simulink model "ACC_demo"  (R2016a)
settings: Solver=VariableStepAuto  StartTime=0  StopTime=30  MaxStep=0.3  RelTol=1e-5
values from neighbouring files (symbols this model uses):
  gearRatio = 15.0    [ACC_dict.sldd]
  initialVelocity = 0.0    [ACC_dict.sldd]
  rollingRadius = 0.3    [ACC_dict.sldd]
libraries: fl_lib x37, nesl_utility x28, sdl_lib x20, sh_lib x7, simulink x1
settings Model: DataDictionary=ACC_dict.sldd  FPTRunName=FPA_Reference  PauseTimes=3  Creator=oskar  LastModifiedBy=Oskar
settings SolverCC: AlgebraicLoopSolver=LineSearch  SolverResetMethod=Robust
settings DataIOCC: SaveFormat=StructureWithTime  ReturnWorkspaceOutputs=on  ReturnWorkspaceOutputsName=spidata
settings HardwareCC: ProdBitPerLong=64  ProdLargestAtomicInteger=Long  ProdLargestAtomicFloat=Double  ProdLongLongMode=on  ProdHWDeviceType=Intel->x86-64  TargetBitPerLong=64  TargetBitPerPointer=64  TargetLongLongMode=on  TargetIntDivRoundTo=Zero  TargetEndianess=LittleEndian  TargetWordSize=64  TargetHWDeviceType=MATLAB Host  ProdEqTarget=off
settings SFSimCC: SimUserSources=protocol.c
settings RTWCC: SystemTargetFile=rsim.tlc  TemplateMakefile=rsim_default_tmf  Description=Rapid Simulation Target  RTWUseSimCustomCode=on  CustomSource=protocol.c  RTWCompilerOptimization=on
settings CodeAppCC: MaxIdLength=95
settings RSimTargetCC: ERTMultiwordTypeDef=System defined  ERTMultiwordLength=256  GeneratePreprocessorConditionals=Use local settings
settings SimscapeCC: SimscapeLogSimulationStatistics=on  SimscapeLogLimitData=off

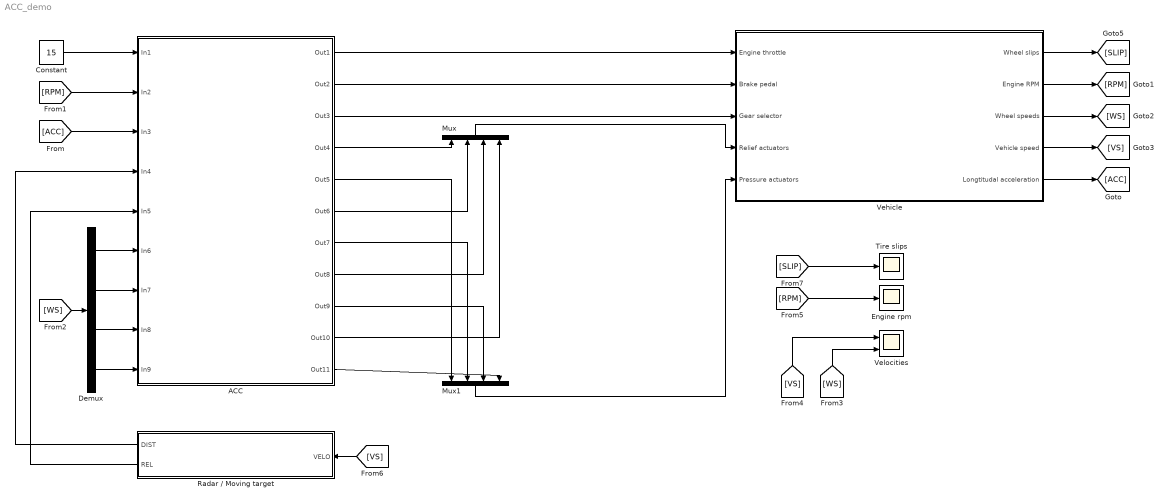
== system ACC_demo ==
  ACC : Subsystem  mask(ARSim){simPath='/Users/Oskar/dev/autosar/arsim-examples/dist/build/acc/acc', numInput=9, numOutput=11}
      mask prompts: simPath "Simulator path"; numInput "# input ports"; numOutput "# output ports"
      mask help:
      | This component acts as an S-function wrapper for the ARSim component. The simulator path parameter needs to be configured as a string pointing to the location of the compiled AUTOSAR component (i.e. with simulateUsingExternal).
      |
      | When the model is initialized, the AUTOSAR simulator will ask for specific port widths. This cannot be adjusted automatically by the Simulink component (yet), so manual intervention is needed, hence the # input/output ports dialogs.
      mask Display: ;port_label('input', 1, 'CRUISE');port_label('input', 2, 'RPM');port_label('input', 3, 'ACCEL');port_label('input', 4, 'DIST');port_label('input', 5, 'REL');port_label('input', 6, 'WHEEL1');port_label('input', 7, 'WHEEL2');port_label('input', 8, 'WHEEL3');port_label('input', 9, 'WHEEL4');port_label('output', 1, 'THR_OUT');port_label('output', 2, 'BRK_OUT');port_label('output', 3, 'GEAR');port_label('output', 4, 'RE');port_label('output', 5, 'PR');port_label('output', 6, 'RE');port_label('output', 7, 'PR');port_label('output', 8, 'RE');port_label('output', 9, 'PR');port_label('output', 10, 'RE');port_label('output', 11, 'PR')
  Constant : Constant  Value=15
  Demux : Demux
  Engine rpm : Scope
  Mux : Mux
  Mux1 : Mux
  Radar / Moving target : Subsystem  mask{dist0=50, velo0=10}
      mask prompts: dist0 "Initial distance"; velo0 "Initial velocity"
  Tire slips : Scope
  Vehicle : Subsystem
  Velocities : Scope  NumInputPorts=2
  wires:
  ACC/4(Out4) -> Mux/1
  ACC/6(Out6) -> Mux/2
  ACC/8(Out8) -> Mux/3
  ACC/10(Out10) -> Mux/4
  ACC/5(Out5) -> Mux1/1
  ACC/7(Out7) -> Mux1/2
  ACC/9(Out9) -> Mux1/3
  ACC/11(Out11) -> Mux1/4
  ACC/1(Out1) -> Vehicle/1(Engine throttle)
  ACC/2(Out2) -> Vehicle/2(Brake pedal)
  ACC/3(Out3) -> Vehicle/3(Gear selector)
  Mux/1 -> Vehicle/4(Relief actuators)
  Mux1/1 -> Vehicle/5(Pressure actuators)
  [ACC] -> ACC/3(In3)
  Vehicle/5(Longtitudal acceleration) -> [ACC]
  Vehicle/2(Engine RPM) -> [RPM]
  [RPM] -> ACC/2(In2)
  Constant/1 -> ACC/1(In1)
  [WS] -> Demux/1
  [WS] -> Velocities/2
  Vehicle/4(Vehicle speed) -> [VS]
  [VS] -> Velocities/1
  [RPM] -> Engine rpm/1
  [SLIP] -> Tire slips/1
  Vehicle/1(Wheel slips) -> [SLIP]
  Vehicle/3(Wheel speeds) -> [WS]
  Radar / Moving target/1(DIST) -> ACC/4(In4)
  Demux/1 -> ACC/6(In6)
  Demux/2 -> ACC/7(In7)
  Demux/3 -> ACC/8(In8)
  Demux/4 -> ACC/9(In9)
  Radar / Moving target/2(REL) -> ACC/5(In5)
  [VS] -> Radar / Moving target/1(VELO)

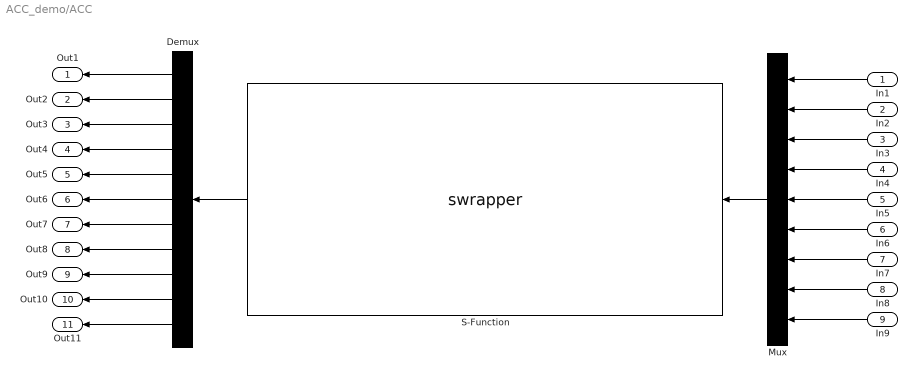
== system ACC_demo/ACC ==
  In1 : Inport  PortDimensions=1
  In2 : Inport  Port=2  PortDimensions=1
  In3 : Inport  Port=3  PortDimensions=1
  In4 : Inport  Port=4  PortDimensions=1
  In5 : Inport  Port=5  PortDimensions=1
  In6 : Inport  Port=6  PortDimensions=1
  In7 : Inport  Port=7  PortDimensions=1
  In8 : Inport  Port=8  PortDimensions=1
  In9 : Inport  Port=9  PortDimensions=1
  Demux : Demux  Outputs=numOutput
  Mux : Mux  Inputs=numInput
  S-Function : S-Function  FunctionName=swrapper  Parameters=simPath  SFunctionDeploymentMode=off  EnableBusSupport=off
  Out1 : Outport  PortDimensions=1
  Out2 : Outport  Port=2  PortDimensions=1
  Out3 : Outport  Port=3  PortDimensions=1
  Out4 : Outport  Port=4  PortDimensions=1
  Out5 : Outport  Port=5  PortDimensions=1
  Out6 : Outport  Port=6  PortDimensions=1
  Out7 : Outport  Port=7  PortDimensions=1
  Out8 : Outport  Port=8  PortDimensions=1
  Out9 : Outport  Port=9  PortDimensions=1
  Out10 : Outport  Port=10  PortDimensions=1
  Out11 : Outport  Port=11  PortDimensions=1
  wires:
  In1/1 -> Mux/1
  Mux/1 -> S-Function/1
  In2/1 -> Mux/2
  S-Function/1 -> Demux/1
  Demux/1 -> Out1/1
  Demux/2 -> Out2/1
  In3/1 -> Mux/3
  In4/1 -> Mux/4
  In5/1 -> Mux/5
  In6/1 -> Mux/6
  Demux/3 -> Out3/1
  In7/1 -> Mux/7
  Demux/11 -> Out11/1
  Demux/10 -> Out10/1
  Demux/9 -> Out9/1
  Demux/8 -> Out8/1
  Demux/7 -> Out7/1
  Demux/6 -> Out6/1
  Demux/5 -> Out5/1
  Demux/4 -> Out4/1
  In8/1 -> Mux/8
  In9/1 -> Mux/9

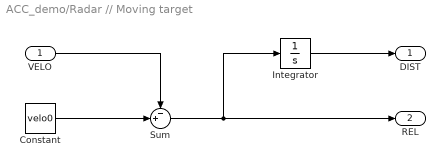
== system ACC_demo/Radar // Moving target ==
  VELO : Inport
  Constant : Constant  Value=velo0
  Integrator : Integrator  InitialCondition=dist0
  Sum : Sum  Inputs=-+|
  DIST : Outport
  REL : Outport  Port=2
  wires:
  Integrator/1 -> DIST/1
  VELO/1 -> Sum/1
  Constant/1 -> Sum/2
  Sum/1 -> Integrator/1, REL/1

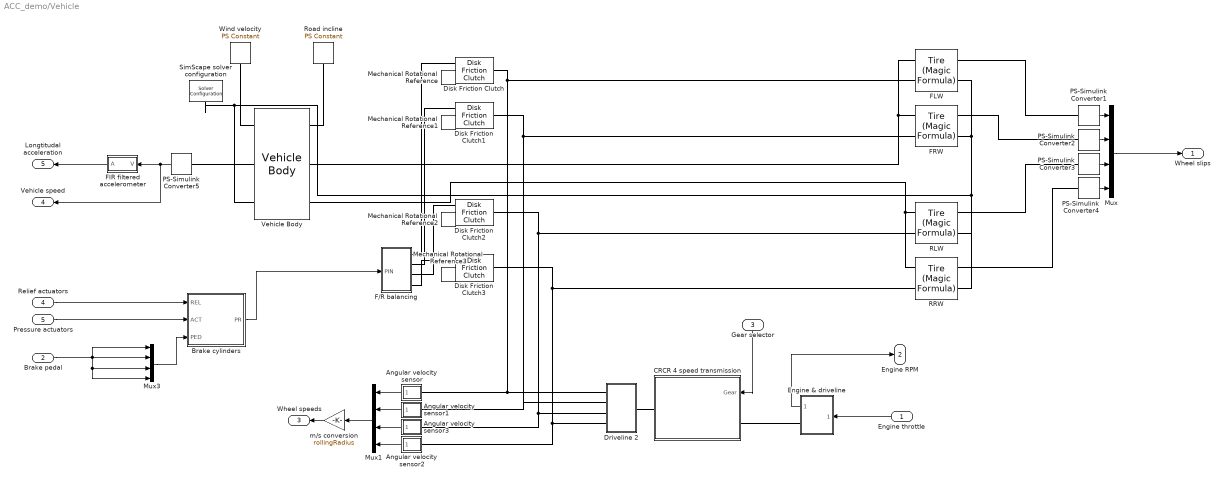
== system ACC_demo/Vehicle ==
  Engine throttle : Inport
  Brake pedal : Inport  Port=2
  Gear selector : Inport  Port=3
  Relief actuators : Inport  Port=4
  Pressure actuators : Inport  Port=5
  Angular velocity sensor : Subsystem
  Angular velocity sensor1 : Subsystem
  Angular velocity sensor2 : Subsystem
  Angular velocity sensor3 : Subsystem
  Brake cylinders : Subsystem  TreatAsAtomicUnit=on
  CRCR 4 speed transmission : Subsystem  mask{ShowInLibBrowser=0}
      settings: OpenFcn=open_system(gcb,'force');
  Disk Friction Clutch{,1..3} (4 alike) : sdl_lib/Clutches/Disk Friction Clutch  geometry_model=1  r_eff=torqueRadius mm  d_o=150 mm  d_i=100 mm  nS=numSurf  piston_area=pistonArea m^2  unidirectional=0  friction_model=1  mu_coulomb=clutchKineticF  mu_w_vector=[ 0 0.1 0.2 0.3 0.4 0.5 1 2 5 10 100 1000 ] rad/s  mu_coulomb_vector=[ 0.29 0.28 0.26 0.22 0.21 0.2 0.2 0.19 0.19 0.19 0.19 0.19 ]  mu_interp_method=1  mu_extrap_method=1  mu_static=clutchStaticF  d_f=1  w_tol=clutchVeloTolRads rad/s  pressure_min=clutchPressureTresh Pa  mu_visc=0 N*m/(rad/s)  initial_state_locked=0
  Driveline 2 : Subsystem
  Engine & driveline : Subsystem
  F/R balancing : Subsystem  mask(F/R Balance){RGain=0.7}
      mask prompts: RGain "Rear pressure gain"
      mask help: Scale the amount of pressure directed to the rear wheels by a constant factor (default 0.7).
  FIR filtered accelerometer : Subsystem
  FLW : sdl_lib/Tires & Vehicles/Tire (Magic Formula)  parameterization=1  F_z1=3e+3 N  F_x1=3.5e+3 N  kappa1=10  B_m=10  C_m=1.9  D_m=1  E_m=0.97  fz0=4e+3 N  p_Cx=1.685  p_Dx=[ 1.21 -0.037 ]  p_Ex=[ 0.344 0.095 -0.02 0 ]  p_Kx=[ 21.51 -0.163 0.245 ]  p_Hx=[ -0.002 0.002 ]  p_Vx=[ 0 0 ]  v_tr_thr=0.1 m/s  r_e=rollingRadius m  model_compliance=0  stiffness=1e+6 N/m  damping=1000 N/(m/s)  model_inertia=0  inertia=1 kg*m^2  initial_velocity=0 rad/s  model_resistance=0  resistance_model=1  coeff=0.015  p_tire=250e3 Pa  alpha=-0.003  beta=0.97  coeff_a=84e-4  coeff_b=6.2e-4 s/m  coeff_c=1.6e-4 s^2/m^2  v_thr=1e-3 m/s
  FRW : sdl_lib/Tires & Vehicles/Tire (Magic Formula)  parameterization=1  F_z1=3e+3 N  F_x1=3.5e+3 N  kappa1=10  B_m=10  C_m=1.9  D_m=1  E_m=0.97  fz0=4e+3 N  p_Cx=1.685  p_Dx=[ 1.21 -0.037 ]  p_Ex=[ 0.344 0.095 -0.02 0 ]  p_Kx=[ 21.51 -0.163 0.245 ]  p_Hx=[ -0.002 0.002 ]  p_Vx=[ 0 0 ]  v_tr_thr=0.1 m/s  r_e=rollingRadius m  model_compliance=0  stiffness=1e+6 N/m  damping=1000 N/(m/s)  model_inertia=0  inertia=1 kg*m^2  initial_velocity=0 rad/s  model_resistance=0  resistance_model=1  coeff=0.015  p_tire=250e3 Pa  alpha=-0.003  beta=0.97  coeff_a=84e-4  coeff_b=6.2e-4 s/m  coeff_c=1.6e-4 s^2/m^2  v_thr=1e-3 m/s
  Mechanical Rotational Reference{,1..3} (4 alike) : fl_lib/Mechanical/Rotational Elements/Mechanical Rotational Reference
  Mux : Mux
  Mux1 : Mux
  Mux3 : Mux
  PS-Simulink Converter{1..5} (5 alike) : nesl_utility/PS-Simulink Converter  PhysicalDomain=network_engine_domain  SubClassName=ps_output  LeftPortType=input  RightPortType=output  PseudoPeriodic=off  Frequencies=[]  Unit=1  AffineConversion=off
  RLW : sdl_lib/Tires & Vehicles/Tire (Magic Formula)  parameterization=1  F_z1=3e+3 N  F_x1=3.5e+3 N  kappa1=10  B_m=10  C_m=1.9  D_m=1  E_m=0.97  fz0=4e+3 N  p_Cx=1.685  p_Dx=[ 1.21 -0.037 ]  p_Ex=[ 0.344 0.095 -0.02 0 ]  p_Kx=[ 21.51 -0.163 0.245 ]  p_Hx=[ -0.002 0.002 ]  p_Vx=[ 0 0 ]  v_tr_thr=0.1 m/s  r_e=rollingRadius m  model_compliance=0  stiffness=1e+6 N/m  damping=1000 N/(m/s)  model_inertia=0  inertia=1 kg*m^2  initial_velocity=0 rad/s  model_resistance=0  resistance_model=1  coeff=0.015  p_tire=250e3 Pa  alpha=-0.003  beta=0.97  coeff_a=84e-4  coeff_b=6.2e-4 s/m  coeff_c=1.6e-4 s^2/m^2  v_thr=1e-3 m/s
  RRW : sdl_lib/Tires & Vehicles/Tire (Magic Formula)  parameterization=1  F_z1=3e+3 N  F_x1=3.5e+3 N  kappa1=10  B_m=10  C_m=1.9  D_m=1  E_m=0.97  fz0=4e+3 N  p_Cx=1.685  p_Dx=[ 1.21 -0.037 ]  p_Ex=[ 0.344 0.095 -0.02 0 ]  p_Kx=[ 21.51 -0.163 0.245 ]  p_Hx=[ -0.002 0.002 ]  p_Vx=[ 0 0 ]  v_tr_thr=0.1 m/s  r_e=rollingRadius m  model_compliance=0  stiffness=1e+6 N/m  damping=1000 N/(m/s)  model_inertia=0  inertia=1 kg*m^2  initial_velocity=0 rad/s  model_resistance=0  resistance_model=1  coeff=0.015  p_tire=250e3 Pa  alpha=-0.003  beta=0.97  coeff_a=84e-4  coeff_b=6.2e-4 s/m  coeff_c=1.6e-4 s^2/m^2  v_thr=1e-3 m/s
  Road incline : fl_lib/Physical Signals/Sources/PS Constant  constant=0
  SimScape solver configuration : nesl_utility/Solver Configuration  PhysicalDomain=network_engine_domain  SubClassName=solver  LeftPortType=input  RightPortType=generic  Accelerate=off  Tones=[]  Harmonics=[]  SimulateNoise=off  Profile=off  UseLocalSampling=off  EnableSwitchedLinearOptims=on  FrequencyDomain=off  UseCCode=off  RelTol=0.001  AbsTol=1e-06  MinStep=1e-09  ToWorkspace=off  RevertToSquareIcSolve=off  NumHomotopyIterations=100  PhasorMode=off  PhasorModeNumHarmonics=1  OverrideAbsTol=off  DoDC=off  ResidualTolerance=1e-09  UseLocalSolver=off  LocalSolverChoice=NE_TRAPEZOIDAL_ADVANCER  LocalSolverSampleTime=0.001  DoFixedCost=off  MaxNonlinIter=3  MaxModeIter=2  LinearAlgebra=Sparse  DelaysMemoryBudget=1024  AutomaticFiltering=on  FilteringTimeConstant=0.001
  Vehicle Body : sdl_lib/Tires & Vehicles/Vehicle Body  mass=1500 kg  n_w=2  x_f=1.4 m  x_r=1.6 m  y_c=0.5 m  area=4 m^2  Cd=0.4  v0=initialVelocity m/s
  Wind velocity : fl_lib/Physical Signals/Sources/PS Constant  constant=10
  m/s conversion : Gain  Gain=rollingRadius
  Wheel slips : Outport
  Engine RPM : Outport  Port=2
  Wheel speeds : Outport  Port=3
  Vehicle speed : Outport  Port=4
  Longtitudal acceleration : Outport  Port=5
  wires:
  m/s conversion/1 -> Wheel speeds/1
  PS-Simulink Converter4/1 -> Mux/4
  PS-Simulink Converter1/1 -> Mux/1
  Mux/1 -> Wheel slips/1
  PS-Simulink Converter2/1 -> Mux/2
  PS-Simulink Converter3/1 -> Mux/3
  Pressure actuators/1 -> Brake cylinders/2(ACT)
  Mux1/1 -> m/s conversion/1
  Engine throttle/1 -> Engine & driveline/1(Throttle)
  Relief actuators/1 -> Brake cylinders/1(REL)
  Angular velocity sensor/1(Out1) -> Mux1/1
  Angular velocity sensor3/1(Out1) -> Mux1/3
  Angular velocity sensor1/1(Out1) -> Mux1/2
  Angular velocity sensor2/1(Out1) -> Mux1/4
  Mux3/1 -> Brake cylinders/3(PED)
  Brake pedal/1 -> Mux3/4, Mux3/3, Mux3/2, Mux3/1
  Brake cylinders/1(PR) -> F/R balancing/1(PIN)
  Engine & driveline/1(rpm) -> Engine RPM/1
  Gear selector/1 -> CRCR 4 speed transmission/1(Gear)
  FIR filtered accelerometer/1(A) -> Longtitudal acceleration/1
  PS-Simulink Converter5/1 -> Vehicle speed/1, FIR filtered accelerometer/1(V)
  connections:
  PS-Simulink Converter4/LConn1 -- RRW/RConn1
  CRCR 4 speed transmission/RConn1 -- Driveline 2/RConn1
  PS-Simulink Converter3/LConn1 -- RLW/RConn1
  PS-Simulink Converter2/LConn1 -- FRW/RConn1
  PS-Simulink Converter1/LConn1 -- FLW/RConn1
  Vehicle Body/RConn1 -- RRW/LConn1 -- RLW/LConn1
  Vehicle Body/RConn2 -- FLW/LConn1 -- FRW/LConn1
  Wind velocity/RConn1 -- Vehicle Body/LConn3
  Vehicle Body/LConn1 -- FLW/RConn2 -- FRW/RConn2 -- RLW/RConn2 -- RRW/RConn2 -- SimScape solver configuration/RConn1
  Road incline/RConn1 -- Vehicle Body/RConn3
  Angular velocity sensor3/LConn1 -- Driveline 2/LConn3 -- Disk Friction Clutch2/RConn1 -- RLW/LConn2
  Disk Friction Clutch1/RConn1 -- Angular velocity sensor1/LConn1 -- Driveline 2/LConn2 -- FRW/LConn2
  Angular velocity sensor/LConn1 -- Disk Friction Clutch/RConn1 -- FLW/LConn2 -- Driveline 2/LConn1
  Angular velocity sensor2/LConn1 -- Driveline 2/LConn4 -- Disk Friction Clutch3/RConn1 -- RRW/LConn2
  Mechanical Rotational Reference/LConn1 -- Disk Friction Clutch/LConn2
  Mechanical Rotational Reference2/LConn1 -- Disk Friction Clutch2/LConn2
  Mechanical Rotational Reference1/LConn1 -- Disk Friction Clutch1/LConn2
  Mechanical Rotational Reference3/LConn1 -- Disk Friction Clutch3/LConn2
  Disk Friction Clutch/LConn1 -- F/R balancing/RConn1
  Disk Friction Clutch1/LConn1 -- F/R balancing/RConn2
  Disk Friction Clutch2/LConn1 -- F/R balancing/RConn3
  Disk Friction Clutch3/LConn1 -- F/R balancing/RConn4
  Engine & driveline/RConn1 -- CRCR 4 speed transmission/LConn1
  PS-Simulink Converter5/LConn1 -- Vehicle Body/LConn2

== system ACC_demo/Vehicle/Angular velocity sensor ==
  PS-Simulink Converter3 : nesl_utility/PS-Simulink Converter  PhysicalDomain=network_engine_domain  SubClassName=ps_output  LeftPortType=input  RightPortType=output  PseudoPeriodic=off  Frequencies=[]  Unit=1  AffineConversion=off
  Reference : fl_lib/Mechanical/Rotational Elements/Mechanical Rotational Reference
  Rotational Motion Sensor : fl_lib/Mechanical/Mechanical Sensors/Ideal Rotational Motion Sensor  offset=0 rad
  Axle : PMIOPort  Port=1  Side=Left
  Out1 : Outport
  wires:
  PS-Simulink Converter3/1 -> Out1/1
  connections:
  Axle/RConn1 -- Rotational Motion Sensor/LConn1
  Reference/LConn1 -- Rotational Motion Sensor/RConn1
  Rotational Motion Sensor/RConn2 -- PS-Simulink Converter3/LConn1

== system ACC_demo/Vehicle/Angular velocity sensor1 ==
  PS-Simulink Converter3 : nesl_utility/PS-Simulink Converter  PhysicalDomain=network_engine_domain  SubClassName=ps_output  LeftPortType=input  RightPortType=output  PseudoPeriodic=off  Frequencies=[]  Unit=1  AffineConversion=off
  Reference : fl_lib/Mechanical/Rotational Elements/Mechanical Rotational Reference
  Rotational Motion Sensor : fl_lib/Mechanical/Mechanical Sensors/Ideal Rotational Motion Sensor  offset=0 rad
  Axle : PMIOPort  Port=1  Side=Left
  Out1 : Outport
  wires:
  PS-Simulink Converter3/1 -> Out1/1
  connections:
  Axle/RConn1 -- Rotational Motion Sensor/LConn1
  Reference/LConn1 -- Rotational Motion Sensor/RConn1
  Rotational Motion Sensor/RConn2 -- PS-Simulink Converter3/LConn1

== system ACC_demo/Vehicle/Angular velocity sensor2 ==
  PS-Simulink Converter3 : nesl_utility/PS-Simulink Converter  PhysicalDomain=network_engine_domain  SubClassName=ps_output  LeftPortType=input  RightPortType=output  PseudoPeriodic=off  Frequencies=[]  Unit=1  AffineConversion=off
  Reference : fl_lib/Mechanical/Rotational Elements/Mechanical Rotational Reference
  Rotational Motion Sensor : fl_lib/Mechanical/Mechanical Sensors/Ideal Rotational Motion Sensor  offset=0 rad
  Axle : PMIOPort  Port=1  Side=Left
  Out1 : Outport
  wires:
  PS-Simulink Converter3/1 -> Out1/1
  connections:
  Axle/RConn1 -- Rotational Motion Sensor/LConn1
  Reference/LConn1 -- Rotational Motion Sensor/RConn1
  Rotational Motion Sensor/RConn2 -- PS-Simulink Converter3/LConn1

== system ACC_demo/Vehicle/Angular velocity sensor3 ==
  PS-Simulink Converter3 : nesl_utility/PS-Simulink Converter  PhysicalDomain=network_engine_domain  SubClassName=ps_output  LeftPortType=input  RightPortType=output  PseudoPeriodic=off  Frequencies=[]  Unit=1  AffineConversion=off
  Reference : fl_lib/Mechanical/Rotational Elements/Mechanical Rotational Reference
  Rotational Motion Sensor : fl_lib/Mechanical/Mechanical Sensors/Ideal Rotational Motion Sensor  offset=0 rad
  Axle : PMIOPort  Port=1  Side=Left
  Out1 : Outport
  wires:
  PS-Simulink Converter3/1 -> Out1/1
  connections:
  Axle/RConn1 -- Rotational Motion Sensor/LConn1
  Reference/LConn1 -- Rotational Motion Sensor/RConn1
  Rotational Motion Sensor/RConn2 -- PS-Simulink Converter3/LConn1

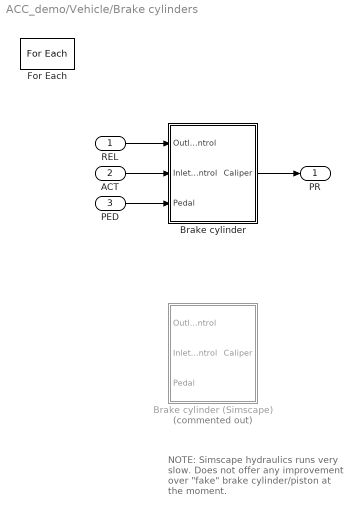
== system ACC_demo/Vehicle/Brake cylinders ==
  note: NOTE: Simscape hydraulics
      | runs very slow. Does not offer
      | any improvement over "fake"
      | brake cylinder/piston at the
      | moment.
  REL : Inport  Partition=on  PartitionDimension=1  PartitionWidth=1
  ACT : Inport  Port=2  Partition=on  PartitionDimension=1  PartitionWidth=1
  PED : Inport  Port=3  Partition=on  PartitionDimension=1  PartitionWidth=1
  Brake cylinder : Subsystem
  Brake cylinder (Simscape) : Subsystem  Commented=on
  For Each : ForEach  DisableCoverage=on  IndexMode=One-based
  PR : Outport  Unit=Pa  ConcatenationDimension=1
  wires:
  Brake cylinder/1(Caliper) -> PR/1
  REL/1 -> Brake cylinder/1(Outlet control)
  ACT/1 -> Brake cylinder/2(Inlet control)
  PED/1 -> Brake cylinder/3(Pedal)

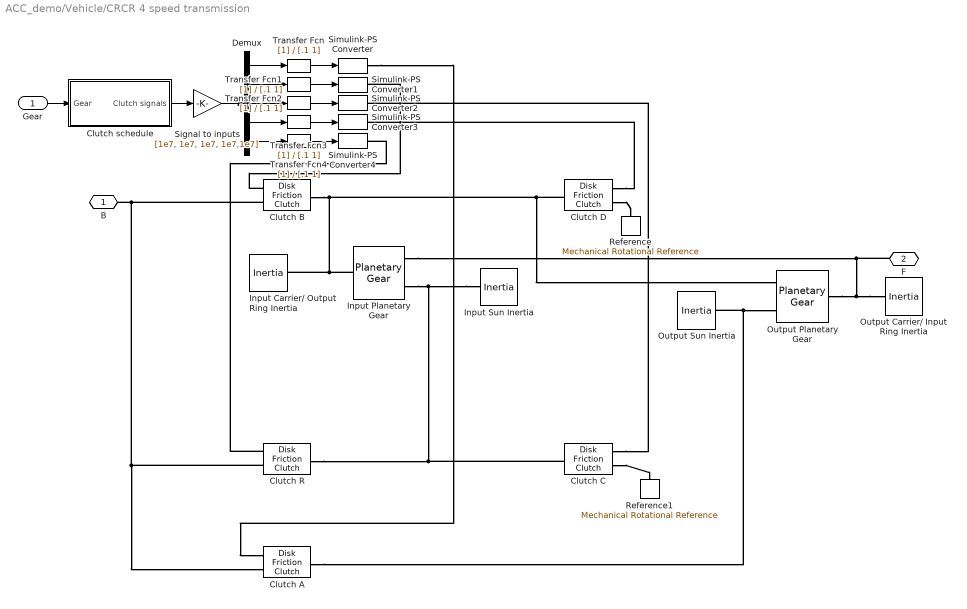
== system ACC_demo/Vehicle/CRCR 4 speed transmission ==
  Gear : Inport
  Clutch A : sdl_lib/Clutches/Disk Friction Clutch  geometry_model=1  r_eff=.05 m  d_o=0.15 m  d_i=0.1 m  nS=6  piston_area=1e-3 m^2  unidirectional=0  friction_model=1  mu_coulomb=.5  mu_w_vector=[ 0 0.1 0.2 0.3 0.4 0.5 1 2 5 10 100 1000 ] rad/s  mu_coulomb_vector=[ 0.29 0.28 0.26 0.22 0.21 0.2 0.2 0.19 0.19 0.19 0.19 0.19 ]  mu_interp_method=1  mu_extrap_method=1  mu_static=.55  d_f=1  w_tol=1e-3 rad/s  pressure_min=1e4 Pa  mu_visc=0 N*m/(rad/s)  initial_state_locked=1
  Clutch B : sdl_lib/Clutches/Disk Friction Clutch  geometry_model=1  r_eff=.05 m  d_o=0.15 m  d_i=0.1 m  nS=6  piston_area=1e-3 m^2  unidirectional=0  friction_model=1  mu_coulomb=.5  mu_w_vector=[ 0 0.1 0.2 0.3 0.4 0.5 1 2 5 10 100 1000 ] rad/s  mu_coulomb_vector=[ 0.29 0.28 0.26 0.22 0.21 0.2 0.2 0.19 0.19 0.19 0.19 0.19 ]  mu_interp_method=1  mu_extrap_method=1  mu_static=.55  d_f=1  w_tol=1e-3 rad/s  pressure_min=1e4 Pa  mu_visc=0 N*m/(rad/s)  initial_state_locked=0
  Clutch C : sdl_lib/Clutches/Disk Friction Clutch  geometry_model=1  r_eff=.05 m  d_o=0.15 m  d_i=0.1 m  nS=6  piston_area=1e-3 m^2  unidirectional=0  friction_model=1  mu_coulomb=.5  mu_w_vector=[ 0 0.1 0.2 0.3 0.4 0.5 1 2 5 10 100 1000 ] rad/s  mu_coulomb_vector=[ 0.29 0.28 0.26 0.22 0.21 0.2 0.2 0.19 0.19 0.19 0.19 0.19 ]  mu_interp_method=1  mu_extrap_method=1  mu_static=.55  d_f=1  w_tol=1e-3 rad/s  pressure_min=1e4 Pa  mu_visc=0 N*m/(rad/s)  initial_state_locked=0
  Clutch D : sdl_lib/Clutches/Disk Friction Clutch  geometry_model=1  r_eff=.05 m  d_o=0.15 m  d_i=0.1 m  nS=6  piston_area=1e-3 m^2  unidirectional=0  friction_model=1  mu_coulomb=.5  mu_w_vector=[ 0 0.1 0.2 0.3 0.4 0.5 1 2 5 10 100 1000 ] rad/s  mu_coulomb_vector=[ 0.29 0.28 0.26 0.22 0.21 0.2 0.2 0.19 0.19 0.19 0.19 0.19 ]  mu_interp_method=1  mu_extrap_method=1  mu_static=.55  d_f=1  w_tol=1e-3 rad/s  pressure_min=1e4 Pa  mu_visc=0 N*m/(rad/s)  initial_state_locked=1
  Clutch R : sdl_lib/Clutches/Disk Friction Clutch  geometry_model=1  r_eff=.05 m  d_o=0.15 m  d_i=0.1 m  nS=6  piston_area=1e-3 m^2  unidirectional=0  friction_model=1  mu_coulomb=.5  mu_w_vector=[ 0 0.1 0.2 0.3 0.4 0.5 1 2 5 10 100 1000 ] rad/s  mu_coulomb_vector=[ 0.29 0.28 0.26 0.22 0.21 0.2 0.2 0.19 0.19 0.19 0.19 0.19 ]  mu_interp_method=1  mu_extrap_method=1  mu_static=.55  d_f=1  w_tol=1e-3 rad/s  pressure_min=1e4 Pa  mu_visc=0 N*m/(rad/s)  initial_state_locked=0
  Clutch schedule : Subsystem
  Demux : Demux  Outputs=5
  "Input Planetary Gear " : sdl_lib/Gears/Planetary Gear  rs_ratio=2  friction_model=1  efficiency=[ 0.96 0.98 ]  mu_visc=[ 0 0 ] N*m/(rad/s)  pwr_thr=[ 0.001 0.001 ] W  planet_inertia=0 kg*m^2  temperature_TLU=[ 280 300 320 ] K  efficiency_sp_TLU=[ 0.95 0.9 0.85 ]  efficiency_rp_TLU=[ 0.95 0.9 0.85 ]  thermal_mass=50 J/K  T_init=300 K
  Input Sun Inertia : fl_lib/Mechanical/Rotational Elements/Inertia  inertia=1e-4 kg*m^2  w_specify=on  w_priority=High  w=0 rad/s  t_specify=off  t_priority=High  t=0 N*m
  Input Carrier/ Output Ring Inertia : fl_lib/Mechanical/Rotational Elements/Inertia  inertia=1e-4 kg*m^2  w_specify=off  w_priority=High  w=initialVelocity/rollingRadius rad/s  t_specify=off  t_priority=High  t=0 N*m
  Output Planetary Gear : sdl_lib/Gears/Planetary Gear  rs_ratio=2  friction_model=1  efficiency=[ 0.96 0.98 ]  mu_visc=[ 0 0 ] N*m/(rad/s)  pwr_thr=[ 0.001 0.001 ] W  planet_inertia=0 kg*m^2  temperature_TLU=[ 280 300 320 ] K  efficiency_sp_TLU=[ 0.95 0.9 0.85 ]  efficiency_rp_TLU=[ 0.95 0.9 0.85 ]  thermal_mass=50 J/K  T_init=300 K
  Output Sun Inertia : fl_lib/Mechanical/Rotational Elements/Inertia  inertia=1e-4 kg*m^2  w_specify=on  w_priority=High  w=3*gearRatio*initialVelocity/rollingRadius rad/s  t_specify=off  t_priority=High  t=0 N*m
  "Output Carrier/ Input Ring Inertia " : fl_lib/Mechanical/Rotational Elements/Inertia  inertia=1e-4 kg*m^2  w_specify=on  w_priority=Low  w=gearRatio*initialVelocity/rollingRadius rad/s  t_specify=off  t_priority=High  t=0 N*m
  Reference : fl_lib/Mechanical/Rotational Elements/Mechanical Rotational Reference
  Reference1 : fl_lib/Mechanical/Rotational Elements/Mechanical Rotational Reference
  Signal to inputs : Gain  Gain=[1e7, 1e7, 1e7, 1e7,1e7]
  Simulink-PS Converter{,1..4} (5 alike) : nesl_utility/Simulink-PS Converter  PhysicalDomain=network_engine_domain  SubClassName=ps_input  LeftPortType=input  RightPortType=output  PseudoPeriodic=off  Frequencies=[]  NoiseDistribution=none  NoiseParameters=[]  Unit=1  AffineConversion=off  InputFiltering=off  SimscapeFilterOrder=1  InputFilterTimeConstant=0.001  UdotUserProvided=1
  Transfer Fcn{,1..4} (5 alike) : TransferFcn  Denominator=[.1 1]
  B : PMIOPort  Port=1  Side=Left
  F : PMIOPort  Port=2  Side=Right
  wires:
  Transfer Fcn1/1 -> Simulink-PS Converter1/1
  Transfer Fcn2/1 -> Simulink-PS Converter2/1
  Transfer Fcn3/1 -> Simulink-PS Converter3/1
  Transfer Fcn4/1 -> Simulink-PS Converter4/1
  Demux/4 -> Transfer Fcn3/1
  Demux/5 -> Transfer Fcn4/1
  Demux/3 -> Transfer Fcn2/1
  Demux/2 -> Transfer Fcn1/1
  Transfer Fcn/1 -> Simulink-PS Converter/1
  Gear/1 -> Clutch schedule/1(Gear)
  Clutch schedule/1(Clutch signals) -> Signal to inputs/1
  Signal to inputs/1 -> Demux/1
  Demux/1 -> Transfer Fcn/1
  connections:
  "Output Carrier/ Input Ring Inertia "/LConn1 -- "Input Planetary Gear "/RConn1 -- F/RConn1 -- Output Planetary Gear/LConn1
  Output Sun Inertia/LConn1 -- Clutch A/RConn1 -- Output Planetary Gear/RConn2
  Input Sun Inertia/LConn1 -- "Input Planetary Gear "/RConn2 -- Clutch C/RConn1 -- Clutch R/RConn1
  Input Carrier/ Output Ring Inertia/LConn1 -- "Input Planetary Gear "/LConn1 -- Clutch B/RConn1 -- Clutch D/RConn1 -- Output Planetary Gear/RConn1
  Clutch R/LConn2 -- Clutch A/LConn2 -- Clutch B/LConn2 -- B/RConn1
  Clutch D/LConn2 -- Reference/LConn1
  Clutch D/LConn1 -- Simulink-PS Converter3/RConn1
  Clutch C/LConn2 -- Reference1/LConn1
  Clutch R/LConn1 -- Simulink-PS Converter4/RConn1
  Clutch C/LConn1 -- Simulink-PS Converter2/RConn1
  Simulink-PS Converter/RConn1 -- Clutch A/LConn1
  Clutch B/LConn1 -- Simulink-PS Converter1/RConn1

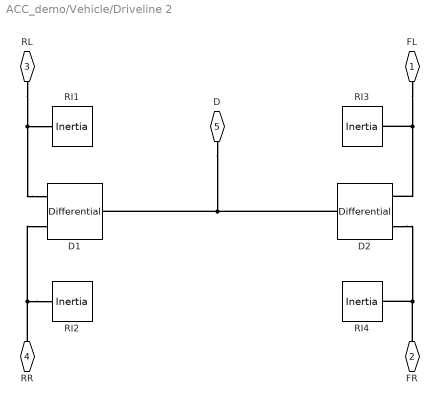
== system ACC_demo/Vehicle/Driveline 2 ==
  D1 : sdl_lib/Gears/Differential  driveshaft_location=2  cd_ratio=gearRatio  friction_model=1  efficiency=[ 0.85 0.92 ]  mu_visc=[ 0 0 ] N*m/(rad/s)  pwr_thr=[ 0.001 0.001 ] W  carrier_inertia=0 kg*m^2  planet_inertia=0 kg*m^2  temperature_TLU=[ 280 300 320 ] K  efficiency_ss_TLU=[ 0.95 0.9 0.85 ]  efficiency_cd_TLU=[ 0.95 0.9 0.85 ]  thermal_mass=50 J/K  T_init=300 K
  D2 : sdl_lib/Gears/Differential  driveshaft_location=2  cd_ratio=gearRatio  friction_model=1  efficiency=[ 0.85 0.92 ]  mu_visc=[ 0 0 ] N*m/(rad/s)  pwr_thr=[ 0.001 0.001 ] W  carrier_inertia=0 kg*m^2  planet_inertia=0 kg*m^2  temperature_TLU=[ 280 300 320 ] K  efficiency_ss_TLU=[ 0.95 0.9 0.85 ]  efficiency_cd_TLU=[ 0.95 0.9 0.85 ]  thermal_mass=50 J/K  T_init=300 K
  RI1 : fl_lib/Mechanical/Rotational Elements/Inertia  inertia=axleInertia kg*m^2  w_specify=on  w_priority=High  w=initialVelocity/rollingRadius rad/s  t_specify=off  t_priority=High  t=0 N*m
  RI2 : fl_lib/Mechanical/Rotational Elements/Inertia  inertia=axleInertia kg*m^2  w_specify=on  w_priority=High  w=initialVelocity/rollingRadius rad/s  t_specify=off  t_priority=High  t=0 N*m
  RI3 : fl_lib/Mechanical/Rotational Elements/Inertia  inertia=2 kg*m^2  w_specify=on  w_priority=High  w=initialVelocity/rollingRadius rad/s  t_specify=off  t_priority=High  t=0 N*m
  RI4 : fl_lib/Mechanical/Rotational Elements/Inertia  inertia=2 kg*m^2  w_specify=on  w_priority=High  w=initialVelocity/rollingRadius rad/s  t_specify=off  t_priority=High  t=0 N*m
  FL : PMIOPort  Port=1  Side=Left
  FR : PMIOPort  Port=2  Side=Left
  RL : PMIOPort  Port=3  Side=Left
  RR : PMIOPort  Port=4  Side=Left
  D : PMIOPort  Port=5  Side=Right
  connections:
  D/RConn1 -- D1/LConn1 -- D2/LConn1
  D2/RConn2 -- FR/RConn1 -- RI4/LConn1
  D1/RConn1 -- RI1/LConn1 -- RL/RConn1
  RI3/LConn1 -- D2/RConn1 -- FL/RConn1
  RI2/LConn1 -- RR/RConn1 -- D1/RConn2

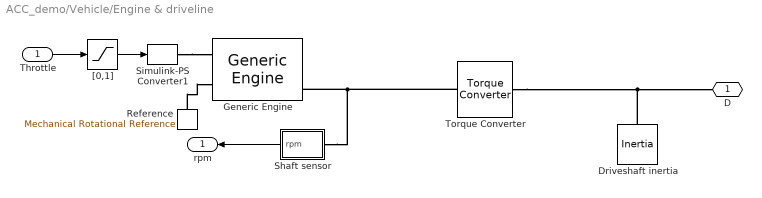
== system ACC_demo/Vehicle/Engine & driveline ==
  Throttle : Inport
  Driveshaft inertia : fl_lib/Mechanical/Rotational Elements/Inertia  inertia=1 kg*m^2  w_specify=on  w_priority=High  w=0 rpm  t_specify=off  t_priority=High  t=0 N*m
  Generic Engine : sdl_lib/Engines/Generic Engine  model_parameterization=1  engine_type=1  P_max=150e3 W  w_P_max=4500 rpm  w_max=6000 rpm  w_min=500 rpm  w_tab=[ 500 1000 2e+3 3e+3 4e+3 5e+3 6e+3 7e+3 ] rpm  trq_tab=[ 380 380 380 380 350 280 200 80 ] N*m  pwr_tab=[ 2e+4 4e+4 7.8e+4 1.2e+5 1.45e+5 1.48e+5 1.25e+5 6e+4 ] W  interp_method=1  model_inertia=1  inertia=0.2 kg*m^2  initial_velocity=1000 rpm  model_time_constant=0  time_constant=0.2 s  T0=0  w_thr=100 rpm  idle_speed=0  idle_speed_reference=1000 rpm  tau_controller=1 s  idle_w_thr=1 rpm  fc_model=1  fc_per_rev=25 mg/rev  displaced_volume=400 cm^3  rev_per_cycle=2  fc_w_tab=[ 1000 2e+3 3e+3 4e+3 5e+3 6e+3 ] rpm  fc_trq_tab=[ 0 80 160 200 240 320 360 400 ] N*m  fc_tab=[ 0.5 0.9 1.4 1.6 1.9 2.7 3.4 4.4; 1 1.7 2.7 3.1 3.6 5 6 7.4; 1.4 2.7 4 4.8 5.6 7.5 8.5 10.5; 2 3.6 5.8 6.7 8 10.4 11.7 13.3; 2.5 4.8 7.9 9.4 10.8 14 16.2 18.6; 3.1 6 10.3 11.9 13.8 18.4 22 26.5 ] g/s  bmep_tab=[ 0 250 500 625 750 1000 1.15e+3 1.25e+3 ] kPa  bsfc_tab=[ 410 380 300 280 270 290 320 380; 410 370 290 270 260 270 285 320; 415 380 290 275 265 270 270 300; 420 390 310 290 285 280 280 285; 430 410 340 320 310 300 310 320; 450 430 370 340 330 330 350 380 ] g/hr/kW  fc_interp_method=1
  Reference : fl_lib/Mechanical/Rotational Elements/Mechanical Rotational Reference
  Shaft sensor : Subsystem
  Simulink-PS Converter1 : nesl_utility/Simulink-PS Converter  PhysicalDomain=network_engine_domain  SubClassName=ps_input  LeftPortType=input  RightPortType=output  PseudoPeriodic=off  Frequencies=[]  NoiseDistribution=none  NoiseParameters=[]  Unit=1  AffineConversion=off  InputFiltering=off  SimscapeFilterOrder=1  InputFilterTimeConstant=.001  UdotUserProvided=0
  Torque Converter : sdl_lib/Couplings & Drives/Torque Converter  n_vector=[0 0.50 0.60 0.70 0.80 0.87 0.92 0.94 0.96 0.97]  trq_vector=[2.2320 1.5462 1.4058 1.2746 1.1528 1.0732 1.0192 0.9983 0.9983 0.9983]  cf_vector_parameterization=1  cf_vector_reference_speed=1  cf_vector=[12.2938 12.8588 13.1452 13.6285 14.6163 16.2675 19.3503 22.1046 29.9986 50.00] (rad/s)/(N*m)^0.5  cf_vector_sq=1e-3*[ 6.616 6.048 5.787 5.384 4.681 3.779 2.671 2.047 1.111 0.400] N*m/(rad/s)^2  interp_method=2  extrap_method=2  model_lag=1  tau=0.2 s  initial_trq_ratio=0
  "[0,1]" : Saturate  UpperLimit=1  LowerLimit=-1
  D : PMIOPort  Port=1  Side=Right
  rpm : Outport
  wires:
  Shaft sensor/1(rpm) -> rpm/1
  "[0,1]"/1 -> Simulink-PS Converter1/1
  Throttle/1 -> "[0,1]"/1
  connections:
  Shaft sensor/LConn1 -- Torque Converter/LConn1 -- Generic Engine/RConn3
  Reference/LConn1 -- Generic Engine/LConn2
  Simulink-PS Converter1/RConn1 -- Generic Engine/LConn1
  Driveshaft inertia/LConn1 -- Torque Converter/RConn1 -- D/RConn1

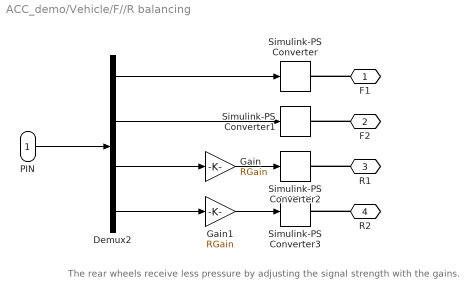
== system ACC_demo/Vehicle/F//R balancing ==
  note: The rear wheels receive less pressure by adjusting the signal strength with the gains.
  PIN : Inport
  Demux2 : Demux
  Gain : Gain  Gain=RGain
  Gain1 : Gain  Gain=RGain
  Simulink-PS Converter{,1..3} (4 alike) : nesl_utility/Simulink-PS Converter  PhysicalDomain=network_engine_domain  SubClassName=ps_input  LeftPortType=input  RightPortType=output  PseudoPeriodic=off  Frequencies=[]  NoiseDistribution=none  NoiseParameters=[]  Unit=Pa  AffineConversion=off  InputFiltering=off  SimscapeFilterOrder=1  InputFilterTimeConstant=0.001  UdotUserProvided=1
  F1 : PMIOPort  Port=1  Side=Right
  F2 : PMIOPort  Port=2  Side=Right
  R1 : PMIOPort  Port=3  Side=Right
  R2 : PMIOPort  Port=4  Side=Right
  wires:
  PIN/1 -> Demux2/1
  Demux2/1 -> Simulink-PS Converter/1
  Demux2/2 -> Simulink-PS Converter1/1
  Demux2/3 -> Gain/1
  Demux2/4 -> Gain1/1
  Gain/1 -> Simulink-PS Converter2/1
  Gain1/1 -> Simulink-PS Converter3/1
  connections:
  F1/RConn1 -- Simulink-PS Converter/RConn1
  F2/RConn1 -- Simulink-PS Converter1/RConn1
  R1/RConn1 -- Simulink-PS Converter2/RConn1
  R2/RConn1 -- Simulink-PS Converter3/RConn1

== system ACC_demo/Vehicle/FIR filtered accelerometer ==
  V : Inport
  Discrete Derivative : simulink/Discrete/Discrete Derivative  gainval=1.0  ICPrevScaledInput=0  OutMin=[]  OutMax=[]  OutDataType=fixdt(1, 16)  OutScaling=2^-10  DoSatur=off
  Discrete FIR Filter : DiscreteFir
  Rate Transition : RateTransition  OutPortSampleTime=1e-3
  A : Outport
  wires:
  V/1 -> Rate Transition/1
  Discrete Derivative/1 -> Discrete FIR Filter/1
  Rate Transition/1 -> Discrete Derivative/1
  Discrete FIR Filter/1 -> A/1

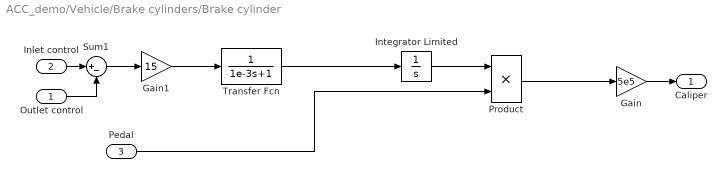
== system ACC_demo/Vehicle/Brake cylinders/Brake cylinder ==
  Outlet control : Inport
  Inlet control : Inport  Port=2
  Pedal : Inport  Port=3
  Gain : Gain  Gain=5e5
  Gain1 : Gain  Gain=15
  Integrator Limited : Integrator  InitialCondition=1  LimitOutput=on  UpperSaturationLimit=1  LowerSaturationLimit=0
  Product : Product
  Sum1 : Sum  Inputs=|+-
  Transfer Fcn : TransferFcn  Denominator=[1e-3 1]
  Caliper : Outport
  wires:
  Gain/1 -> Caliper/1
  Inlet control/1 -> Sum1/1
  Outlet control/1 -> Sum1/2
  Sum1/1 -> Gain1/1
  Pedal/1 -> Product/2
  Gain1/1 -> Transfer Fcn/1
  Transfer Fcn/1 -> Integrator Limited/1
  Integrator Limited/1 -> Product/1
  Product/1 -> Gain/1

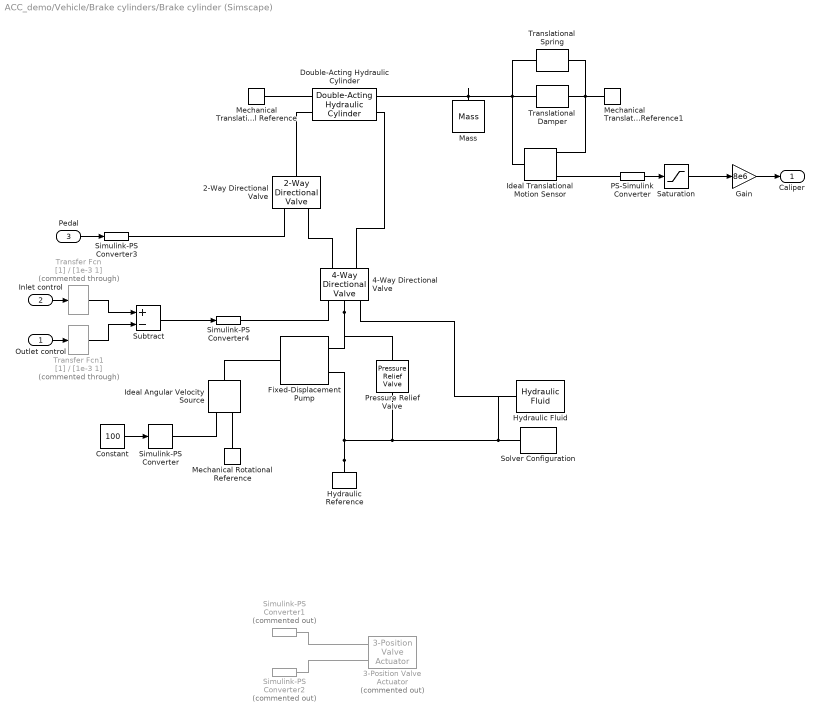
== system ACC_demo/Vehicle/Brake cylinders/Brake cylinder (Simscape) ==
  Outlet control : Inport
  Inlet control : Inport  Port=2
  Pedal : Inport  Port=3
  2-Way Directional Valve : sh_lib/Valves/Directional Valves/2-Way Directional Valve  mdl_type=1  area_max=5e-5 m^2  opening_max=0.005 m  opening_tab=[ -0.002 0 0.002 0.005 0.015 ] m  area_tab=[ 1e-9 2.0352e-7 4.0736e-5 1.1438e-4 3.4356e-4 ] m^2  pressure_tab=[ -1e+7 -5e+6 -2e+6 2e+6 5e+6 1e+7 ] Pa  flow_rate_tab=[ -1e-7 -7.0711e-8 -4.4721e-8 4.4721e-8 7.0711e-8 1e-7; -2.0352e-5 -1.4391e-5 -9.1017e-6 9.1017e-6 1.4391e-5 2.0352e-5; -0.0040736 -0.0028805 -0.0018218 0.0018218 0.0028805 0.0040736; -0.011438 -0.0080879 -0.0051152 0.0051152 0.0080879 0.011438; -0.034356 -0.024293 -0.015364 0.015364 0.024293 0.034356 ] m^3/s  interp_method=1  extrap_method=1  C_d=0.7  x_0=0 m  Re_cr=12  A_leak=1e-12 m^2
  3-Position Valve Actuator : sh_lib/Valves/Valve Actuators/3-Position Valve Actuator  Commented=on  stroke=1 m  t_on=20 ms  t_off=30 ms  act_signal=1  init_position=1
  4-Way Directional Valve : sh_lib/Valves/Directional Valves/4-Way Directional Valve  mdl_type=1  area_max=5e-5 m^2  opening_max=0.005 m  opening_tab=[ -0.002 0 0.002 0.005 0.015 ] m  area_tab=[ 1e-9 2.0352e-7 4.0736e-5 1.1438e-4 3.4356e-4 ] m^2  pressure_tab=[ -1e+7 -5e+6 -2e+6 2e+6 5e+6 1e+7 ] Pa  flow_rate_tab=[ -1e-7 -7.0711e-8 -4.4721e-8 4.4721e-8 7.0711e-8 1e-7; -2.0352e-5 -1.4391e-5 -9.1017e-6 9.1017e-6 1.4391e-5 2.0352e-5; -0.0040736 -0.0028805 -0.0018218 0.0018218 0.0028805 0.0040736; -0.011438 -0.0080879 -0.0051152 0.0051152 0.0080879 0.011438; -0.034356 -0.024293 -0.015364 0.015364 0.024293 0.034356 ] m^3/s  interp_method=1  extrap_method=1  C_d=0.7  x_0_P_A=0 m  x_0_P_B=0 m  x_0_A_T=0 m  x_0_B_T=0 m  Re_cr=12  A_leak=1e-12 m^2
  Constant : Constant  Value=100
  Double-Acting Hydraulic Cylinder : sh_lib/Hydraulic Cylinders/Double-Acting Hydraulic Cylinder  area_A=1e-3 m^2  area_B=0.5e-3 m^2  stroke=0.05 m  init_pos=0 m  dead_vol_A=1e-4 m^3  dead_vol_B=1e-4 m^3  init_pressure_A=0 Pa  init_pressure_B=0 Pa  k_sh=1.4  stiff=1e6 N/m  D=150 N/(m/s)  or=1
  Fixed-Displacement Pump : sh_lib/Pumps and Motors/Fixed-Displacement Pump  D=5e-6 m^3/rad  efficiency_vol=0.92  efficiency_tot=0.8  pr_nominal=100e5 Pa  w_nominal=188 rad/s  visc_nominal=18 cSt  dens_nominal=900 kg/m^3
  Gain : Gain  Gain=8e6
  Hydraulic Fluid : sh_lib/Hydraulic Utilities/Hydraulic Fluid  DataSource=1  SelFluid=19  SysTemp=100  TrapAir=0.005  ViscDerFactor=1  range_error=2
  Hydraulic Reference : fl_lib/Hydraulic/Hydraulic Elements/Hydraulic Reference
  Ideal Angular Velocity Source : fl_lib/Mechanical/Mechanical Sources/Ideal Angular Velocity Source
  Ideal Translational Motion Sensor : fl_lib/Mechanical/Mechanical Sensors/Ideal Translational Motion Sensor  offset=0 m
  Mass : fl_lib/Mechanical/Translational Elements/Mass  mass=0.01 kg  v_specify=off  v_priority=High  v=0 m/s  f_specify=off  f_priority=None  f=0 N
  Mechanical Rotational Reference : fl_lib/Mechanical/Rotational Elements/Mechanical Rotational Reference
  Mechanical Translational Reference : fl_lib/Mechanical/Translational Elements/Mechanical Translational Reference
  Mechanical Translational Reference1 : fl_lib/Mechanical/Translational Elements/Mechanical Translational Reference
  PS-Simulink Converter : nesl_utility/PS-Simulink Converter  PhysicalDomain=network_engine_domain  SubClassName=ps_output  LeftPortType=input  RightPortType=output  PseudoPeriodic=off  Frequencies=[]  Unit=1  AffineConversion=off
  Pressure Relief Valve : sh_lib/Valves/Pressure Control Valves/Pressure Relief Valve  area_max=1e-4 m^2  pres_set=50e5 Pa  reg_range=5e5 Pa  C_d=0.7  Re_cr=12  A_leak=1e-12 m^2  dynamic=0  tau=0.1 s  area_init=1e-12 m^2
  Saturation : Saturate  UpperLimit=0.1  LowerLimit=0
  Simulink-PS Converter : nesl_utility/Simulink-PS Converter  PhysicalDomain=network_engine_domain  SubClassName=ps_input  LeftPortType=input  RightPortType=output  PseudoPeriodic=off  Frequencies=[]  NoiseDistribution=none  NoiseParameters=[]  Unit=1  AffineConversion=off  InputFiltering=off  SimscapeFilterOrder=1  InputFilterTimeConstant=0.001  UdotUserProvided=1
  Simulink-PS Converter1 : nesl_utility/Simulink-PS Converter  Commented=on  PhysicalDomain=network_engine_domain  SubClassName=ps_input  LeftPortType=input  RightPortType=output  PseudoPeriodic=off  Frequencies=[]  NoiseDistribution=none  NoiseParameters=[]  Unit=1  AffineConversion=off  InputFiltering=off  SimscapeFilterOrder=1  InputFilterTimeConstant=0.001  UdotUserProvided=1
  Simulink-PS Converter2 : nesl_utility/Simulink-PS Converter  Commented=on  PhysicalDomain=network_engine_domain  SubClassName=ps_input  LeftPortType=input  RightPortType=output  PseudoPeriodic=off  Frequencies=[]  NoiseDistribution=none  NoiseParameters=[]  Unit=1  AffineConversion=off  InputFiltering=off  SimscapeFilterOrder=1  InputFilterTimeConstant=0.001  UdotUserProvided=1
  Simulink-PS Converter3 : nesl_utility/Simulink-PS Converter  PhysicalDomain=network_engine_domain  SubClassName=ps_input  LeftPortType=input  RightPortType=output  PseudoPeriodic=off  Frequencies=[]  NoiseDistribution=none  NoiseParameters=[]  Unit=1  AffineConversion=off  InputFiltering=off  SimscapeFilterOrder=1  InputFilterTimeConstant=0.001  UdotUserProvided=1
  Simulink-PS Converter4 : nesl_utility/Simulink-PS Converter  PhysicalDomain=network_engine_domain  SubClassName=ps_input  LeftPortType=input  RightPortType=output  PseudoPeriodic=off  Frequencies=[]  NoiseDistribution=none  NoiseParameters=[]  Unit=1  AffineConversion=off  InputFiltering=off  SimscapeFilterOrder=1  InputFilterTimeConstant=0.001  UdotUserProvided=1
  Solver Configuration : nesl_utility/Solver Configuration  PhysicalDomain=network_engine_domain  SubClassName=solver  LeftPortType=input  RightPortType=generic  Accelerate=off  Tones=[]  Harmonics=[]  SimulateNoise=off  Profile=off  UseLocalSampling=off  EnableSwitchedLinearOptims=on  FrequencyDomain=off  UseCCode=off  RelTol=0.001  AbsTol=1e-06  MinStep=1e-09  ToWorkspace=off  RevertToSquareIcSolve=off  NumHomotopyIterations=100  PhasorMode=off  PhasorModeNumHarmonics=1  OverrideAbsTol=off  DoDC=off  ResidualTolerance=1e-09  UseLocalSolver=off  LocalSolverChoice=NE_BACKWARD_EULER_ADVANCER  LocalSolverSampleTime=0.001  DoFixedCost=off  MaxNonlinIter=3  MaxModeIter=2  LinearAlgebra=Sparse  DelaysMemoryBudget=1024  AutomaticFiltering=on  FilteringTimeConstant=0.001
  Subtract : Sum  Inputs=+-
  Transfer Fcn : TransferFcn  Commented=through  Denominator=[1e-3 1]
  Transfer Fcn1 : TransferFcn  Commented=through  Denominator=[1e-3 1]
  Translational Damper : fl_lib/Mechanical/Translational Elements/Translational Damper  D=1 N/(m/s)  v_specify=off  v_priority=None  v=0 m/s  f_specify=off  f_priority=None  f=0 N
  Translational Spring : fl_lib/Mechanical/Translational Elements/Translational Spring  spr_rate=1e2 N/m  v_specify=off  v_priority=None  v=0 m/s  f_specify=off  f_priority=None  f=0 N  x_specify=off  x_priority=High  x=0 m
  Caliper : Outport
  wires:
  PS-Simulink Converter/1 -> Saturation/1
  Pedal/1 -> Simulink-PS Converter3/1
  Constant/1 -> Simulink-PS Converter/1
  Gain/1 -> Caliper/1
  Saturation/1 -> Gain/1
  Outlet control/1 -> Transfer Fcn1/1
  Inlet control/1 -> Transfer Fcn/1
  Subtract/1 -> Simulink-PS Converter4/1
  Transfer Fcn/1 -> Subtract/1
  Transfer Fcn1/1 -> Subtract/2
  connections:
  Translational Spring/LConn1 -- Translational Damper/LConn1 -- Mass/LConn1 -- Double-Acting Hydraulic Cylinder/RConn1 -- Ideal Translational Motion Sensor/LConn1
  Translational Damper/RConn1 -- Mechanical Translational Reference1/LConn1 -- Translational Spring/RConn1 -- Ideal Translational Motion Sensor/RConn1
  Hydraulic Reference/LConn1 -- Fixed-Displacement Pump/RConn2 -- 4-Way Directional Valve/RConn3 -- Hydraulic Fluid/RConn1 -- Solver Configuration/RConn1 -- Pressure Relief Valve/RConn1
  4-Way Directional Valve/RConn2 -- Fixed-Displacement Pump/RConn1 -- Pressure Relief Valve/LConn1
  Simulink-PS Converter4/RConn1 -- 4-Way Directional Valve/RConn1
  Mechanical Translational Reference/LConn1 -- Double-Acting Hydraulic Cylinder/LConn1
  Mechanical Rotational Reference/LConn1 -- Ideal Angular Velocity Source/RConn2
  4-Way Directional Valve/LConn2 -- Double-Acting Hydraulic Cylinder/RConn2
  Simulink-PS Converter/RConn1 -- Ideal Angular Velocity Source/RConn1
  Ideal Angular Velocity Source/LConn1 -- Fixed-Displacement Pump/LConn1
  4-Way Directional Valve/LConn1 -- 2-Way Directional Valve/LConn2
  2-Way Directional Valve/RConn1 -- Double-Acting Hydraulic Cylinder/LConn2
  Simulink-PS Converter3/RConn1 -- 2-Way Directional Valve/LConn1
  Ideal Translational Motion Sensor/RConn3 -- PS-Simulink Converter/LConn1
  3-Position Valve Actuator/LConn1 -- Simulink-PS Converter1/RConn1
  3-Position Valve Actuator/LConn2 -- Simulink-PS Converter2/RConn1

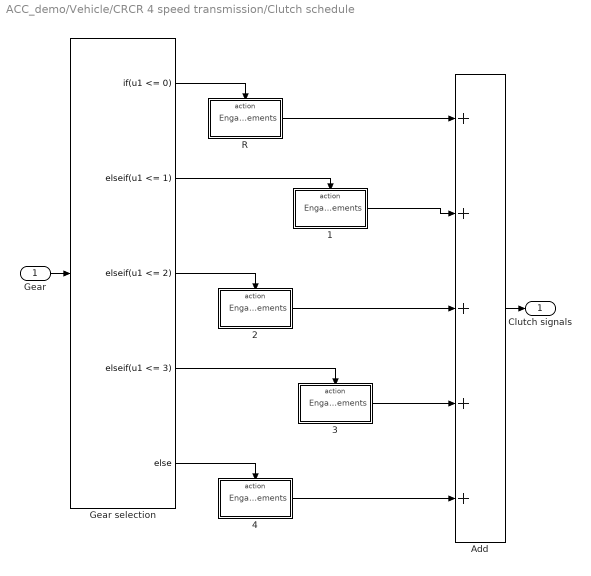
== system ACC_demo/Vehicle/CRCR 4 speed transmission/Clutch schedule ==
  Gear : Inport
  1 : Subsystem  TreatAsAtomicUnit=on
  2 : Subsystem  TreatAsAtomicUnit=on
  3 : Subsystem  TreatAsAtomicUnit=on
  4 : Subsystem  TreatAsAtomicUnit=on
  Add : Sum  Inputs=+++++
  Gear selection : If  IfExpression=u1 <= 0  ElseIfExpressions=u1 <= 1, u1 <= 2, u1 <= 3
  R : Subsystem  TreatAsAtomicUnit=on
  Clutch signals : Outport
  wires:
  Gear selection/5 -> 4/Action
  4/1(Engagements) -> Add/5
  Add/1 -> Clutch signals/1
  Gear/1 -> Gear selection/1
  1/1(Engagements) -> Add/2
  3/1(Engagements) -> Add/4
  2/1(Engagements) -> Add/3
  R/1(Engagements) -> Add/1
  Gear selection/4 -> 3/Action
  Gear selection/3 -> 2/Action
  Gear selection/2 -> 1/Action
  Gear selection/1 -> R/Action

== system ACC_demo/Vehicle/Engine & driveline/Shaft sensor ==
  PS-Simulink Converter3 : nesl_utility/PS-Simulink Converter  PhysicalDomain=network_engine_domain  SubClassName=ps_output  LeftPortType=input  RightPortType=output  PseudoPeriodic=off  Frequencies=[]  Unit=rpm  AffineConversion=off
  Reference : fl_lib/Mechanical/Rotational Elements/Mechanical Rotational Reference
  Rotational Motion Sensor : fl_lib/Mechanical/Mechanical Sensors/Ideal Rotational Motion Sensor  offset=0 rad
  R : PMIOPort  Port=1  Side=Left
  rpm : Outport
  wires:
  PS-Simulink Converter3/1 -> rpm/1
  connections:
  R/RConn1 -- Rotational Motion Sensor/LConn1
  Reference/LConn1 -- Rotational Motion Sensor/RConn1
  Rotational Motion Sensor/RConn2 -- PS-Simulink Converter3/LConn1

== system ACC_demo/Vehicle/CRCR 4 speed transmission/Clutch schedule/1 ==
  Action Port : ActionPort  ActionType=elseif
  Transmission engagements : Constant  Value=[1, 0, 0, 1, 0]
  Engagements : Outport  OutputWhenDisabled=reset  InitialOutput=[0, 0, 0, 0, 0]
  wires:
  Transmission engagements/1 -> Engagements/1

== system ACC_demo/Vehicle/CRCR 4 speed transmission/Clutch schedule/2 ==
  Action Port : ActionPort  ActionType=elseif
  Transmission engagements : Constant  Value=[1, 0, 1, 0, 0]
  Engagements : Outport  OutputWhenDisabled=reset  InitialOutput=[0, 0, 0, 0, 0]
  wires:
  Transmission engagements/1 -> Engagements/1

== system ACC_demo/Vehicle/CRCR 4 speed transmission/Clutch schedule/3 ==
  Action Port : ActionPort  ActionType=elseif
  Transmission engagements : Constant  Value=[1, 1, 0, 0, 0]
  Engagements : Outport  OutputWhenDisabled=reset  InitialOutput=[0, 0, 0, 0, 0]
  wires:
  Transmission engagements/1 -> Engagements/1

== system ACC_demo/Vehicle/CRCR 4 speed transmission/Clutch schedule/4 ==
  Action Port : ActionPort  ActionType=else
  Transmission engagements : Constant  Value=[0, 1, 1, 0, 0]
  Engagements : Outport  OutputWhenDisabled=reset  InitialOutput=[0, 0, 0, 0, 0]
  wires:
  Transmission engagements/1 -> Engagements/1

== system ACC_demo/Vehicle/CRCR 4 speed transmission/Clutch schedule/R ==
  Action Port : ActionPort  ActionType=then
  Transmission engagements : Constant  Value=[0, 0, 0, 0, 0]
  Engagements : Outport  OutputWhenDisabled=reset  InitialOutput=[0, 0, 0, 0, 0]
  wires:
  Transmission engagements/1 -> Engagements/1
